simulink model "Logic"  (R2017a)
settings: Solver=FixedStepDiscrete  StartTime=0.0  StopTime=0.1  FixedStep=2e-6  MaxStep=1e-4  RelTol=1e-3
undefined symbols (not defined in the file): DiscIntNeverNeededParam
libraries: powerlib_meascontrol x1, powerlib x1
settings Model: Creator=mayartmal  LastModifiedBy=mayartmal

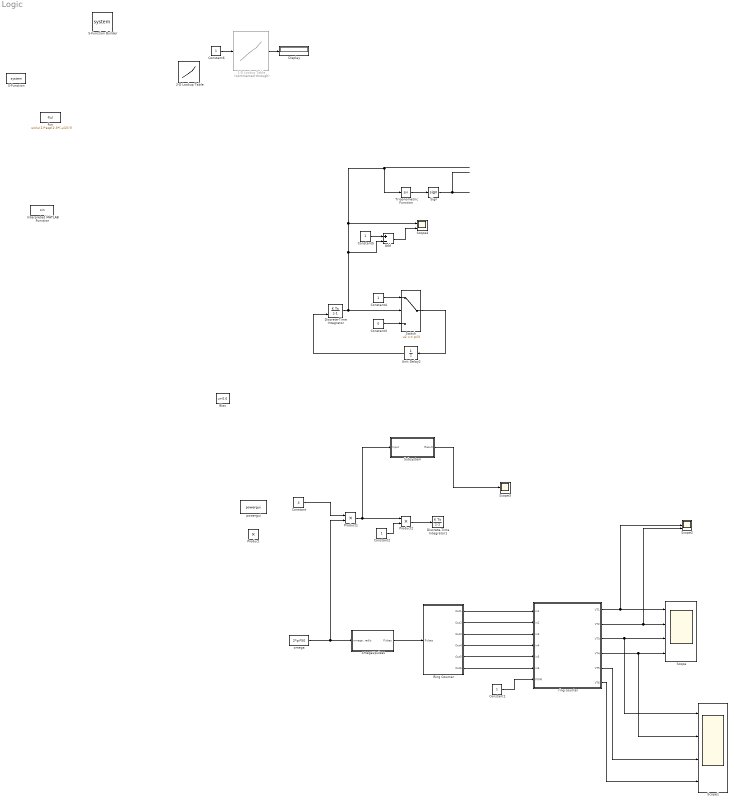
== system Logic ==
  1-D Lookup Table : Lookup_n-D  Commented=through  NumberOfTableDimensions=1  BreakpointsForDimension1=[1:5]  Table=[2:10]  InternalRulePriority=Speed  RndMeth=Simplest  InputSameDT=on
  2-D Lookup Table : Lookup_n-D  BreakpointsForDimension1=[1:3]  BreakpointsForDimension2=[1:3]  InternalRulePriority=Speed  RndMeth=Simplest  InputSameDT=on
  Add : Sum  Inputs=+-
  Bias : Bias  Bias=0.0
  Constant : Constant  Value=4
  Constant{1..2,4..6} (5 alike) : Constant
  Constant3 : Constant  Value=0
  Discrete-Time Integrator : DiscreteIntegrator  gainval=1  ExternalReset=rising  InitialConditionSetting=State (most efficient)  SampleTime=-1  ICPrevOutput=DiscIntNeverNeededParam  ICPrevScaledInput=DiscIntNeverNeededParam
  Discrete-Time Integrator1 : DiscreteIntegrator  gainval=1  InitialConditionSetting=State (most efficient)  SampleTime=-1  ICPrevOutput=DiscIntNeverNeededParam  ICPrevScaledInput=DiscIntNeverNeededParam
  Display : Display
  Fcn : Fcn  Expr=sin(u(1)*exp(2.3*(-u(2))))
  Interpreted MATLAB Function : MATLABFcn
  Product : Product
  Product1 : Product
  Product2 : Product
  Ring Counter : Subsystem
  S-Function : S-Function  SFunctionDeploymentMode=off  EnableBusSupport=off
  S-Function Builder : S-Function  SFunctionDeploymentMode=off  EnableBusSupport=off  mask(S-Function Builder){}
      mask help: Simulink:masks:SFunctionBuilder_MD
      mask init:
      | val = [[.9  0.75 0.75 1 1 .9 .9 1]',[1 1 0.75 0.75 .9 .9 1 .9]'];try , sys = get_param(gcb,'SfunBuilderFcnName');if isempty(sys), sys = get_param(gcb,'FunctionName'); end,catch, sys = get_param(gcb,'FunctionName'); end
      settings: CopyFcn=set_param(gcbh,'LinkStatus','none')  OpenFcn=sfunctionwizard(gcbh)
      mask Display: plot(val(:,1),val(:,2)),disp(sys), port_label('input',1,'u0'), port_label('output',1,'y0')
  Scope : Scope  NumInputPorts=4
  Scope1 : Scope  NumInputPorts=4
  Scope2 : Scope  NumInputPorts=3
  Scope3 : Scope
  Scope4 : Scope  NumInputPorts=2
  Sign : Signum
  Subsystem : Subsystem
  Switch : Switch  Threshold=pi/3
  Trigonometric Function : Trigonometry
  Unit Delay2 : UnitDelay  SampleTime=-1
  omega : Constant  Value=2*pi*50
  omega2pulses : Subsystem
  powergui : powerlib/powergui  Priority=1  SimulationMode=Discrete  SampleTime=2e-6  frequency=60  Iterations=50  frequencyindice=0  Pbase=100e6  ErrMax=1e-4  UnitsV=kV  UnitsW=MW  buscounter=0  FunctionMessages=off  echomessages=off  EnableUseOfTLC=off  CurrentSourceSwitches=off  DisableSnubberDevices=off  DisableRonSwitches=off  DisableVfSwitches=off  DisplayEquations=off  SolverType=Tustin/Backward Euler (TBE)  Interpol=off  ExternalGateDelay=off  methode=off  Ts=100  x0status=blocks  SPID=off  SwTol=0  HookPort=off  RestoreLinks=warning  ResistiveCurrentMeasurement=off  Frange=[0:2:500]  Ylog=off  Xlog=on  ShowGrid=off  save=off  variable=ZData  structure=0  ZoomFFT=off  StartTime=0.0  cycles=1  DisplayStyle=1  fundamental=60  FreqAxis=off  MaxFrequency=1000  frequencyindicesteady=1  RmsSteady=1  display=off
  ring counter : MATLAB Function  TreatAsAtomicUnit=on
  wires:
  omega2pulses/1(Pulses) -> Ring Counter/1(Pulses)
  Constant1/1 -> ring counter/7(PWM)
  ring counter/1(VT1) -> Scope2/2, Scope/1
  Ring Counter/3(Out3) -> ring counter/3(in3)
  Ring Counter/4(Out4) -> ring counter/4(in4)
  Ring Counter/2(Out2) -> ring counter/2(in2)
  Ring Counter/5(Out5) -> ring counter/5(in5)
  Ring Counter/1(Out1) -> ring counter/1(in1)
  Ring Counter/6(Out6) -> ring counter/6(in6)
  ring counter/2(VT2) -> Scope2/3, Scope/2
  ring counter/3(VT3) -> Scope1/1, Scope/3
  ring counter/4(VT4) -> Scope1/2, Scope/4
  ring counter/5(VT5) -> Scope1/3
  ring counter/6(VT6) -> Scope1/4
  omega/1 -> Product1/2, omega2pulses/1("omega, rad/s")
  Constant/1 -> Product1/1
  Discrete-Time Integrator/1 -> Switch/2, Trigonometric Function/1, Scope4/1, Add/2
  Constant5/1 -> Add/1
  Add/1 -> Scope4/2
  Constant3/1 -> Switch/3
  Switch/1 -> Unit Delay2/1
  Constant4/1 -> Switch/1
  Sign/1 -> ?
  Trigonometric Function/1 -> Sign/1
  Unit Delay2/1 -> Discrete-Time Integrator/2
  Product2/1 -> Discrete-Time Integrator1/1
  Product1/1 -> Subsystem/1(Input), Product2/1
  Constant2/1 -> Product2/2
  Subsystem/1(Result) -> Scope3/1
  Constant6/1 -> 1-D Lookup Table/1
  1-D Lookup Table/1 -> Display/1

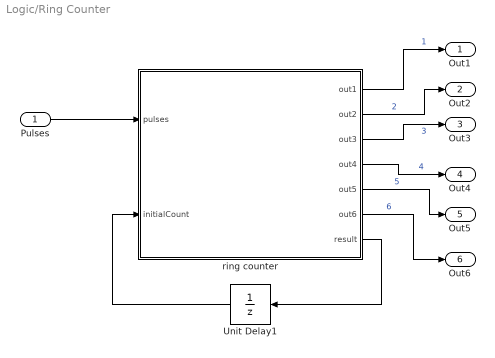
== system Logic/Ring Counter ==
  Pulses : Inport
  Unit Delay1 : UnitDelay  InitialCondition=1  SampleTime=-1
  ring counter : MATLAB Function  TreatAsAtomicUnit=on
  Out1 : Outport
  Out2 : Outport  Port=2
  Out3 : Outport  Port=3
  Out4 : Outport  Port=4
  Out5 : Outport  Port=5
  Out6 : Outport  Port=6
  wires:
  Unit Delay1/1 -> ring counter/2(initialCount)
  ring counter/7(result) -> Unit Delay1/1
  ring counter/3(out3) -> Out3/1  "3"
  ring counter/5(out5) -> Out5/1  "5"
  ring counter/4(out4) -> Out4/1  "4"
  ring counter/2(out2) -> Out2/1  "2"
  ring counter/6(out6) -> Out6/1  "6"
  Pulses/1 -> ring counter/1(pulses)
  ring counter/1(out1) -> Out1/1  "1"

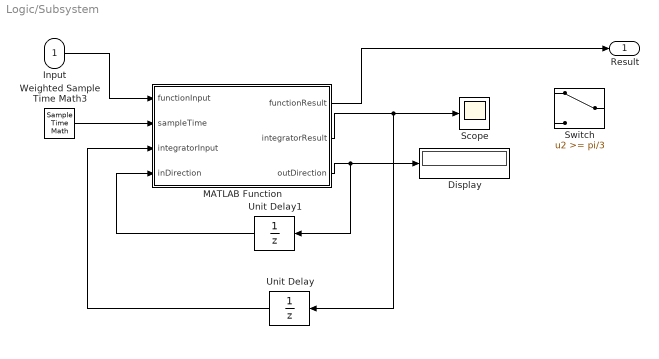
== system Logic/Subsystem ==
  Input : Inport
  Display : Display
  MATLAB Function : MATLAB Function  TreatAsAtomicUnit=on
  Scope : Scope
  Switch : Switch  Threshold=pi/3
  Unit Delay : UnitDelay  SampleTime=-1
  Unit Delay1 : UnitDelay  SampleTime=-1
  Weighted Sample Time Math3 : SampleTimeMath  TsampMathOp=Ts Only
  Result : Outport
  wires:
  Unit Delay/1 -> MATLAB Function/3(integratorInput)
  MATLAB Function/2(integratorResult) -> Scope/1, Unit Delay/1
  MATLAB Function/1(functionResult) -> Result/1
  Weighted Sample Time Math3/1 -> MATLAB Function/2(sampleTime)
  Input/1 -> MATLAB Function/1(functionInput)
  Unit Delay1/1 -> MATLAB Function/4(inDirection)
  MATLAB Function/3(outDirection) -> Unit Delay1/1, Display/1

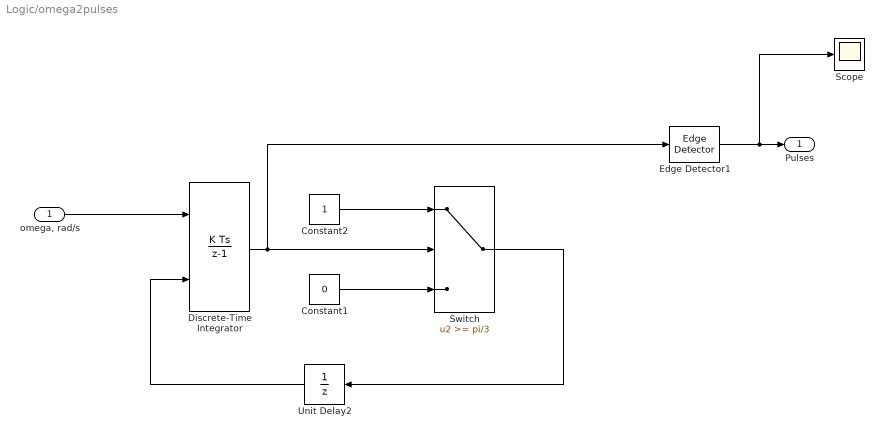
== system Logic/omega2pulses ==
  "omega, rad/s" : Inport
  Constant1 : Constant  Value=0
  Constant2 : Constant
  Discrete-Time Integrator : DiscreteIntegrator  ExternalReset=rising  InitialConditionSetting=State (most efficient)  SampleTime=-1  ICPrevOutput=DiscIntNeverNeededParam  ICPrevScaledInput=DiscIntNeverNeededParam
  Edge Detector1 : powerlib_meascontrol/Logic/Edge Detector  model=Falling  ic=0  Ts=-1
      settings: SourceProductName=Simscape Power Systems  SourceProductBaseCode=PS
  Scope : Scope
  Switch : Switch  Threshold=pi/3
  Unit Delay2 : UnitDelay  SampleTime=-1
  Pulses : Outport
  wires:
  Switch/1 -> Unit Delay2/1
  Discrete-Time Integrator/1 -> Edge Detector1/1, Switch/2
  Unit Delay2/1 -> Discrete-Time Integrator/2
  Constant1/1 -> Switch/3
  Constant2/1 -> Switch/1
  Edge Detector1/1 -> Scope/1, Pulses/1
  "omega, rad/s"/1 -> Discrete-Time Integrator/1

== matlab function Logic/ring counter ==
  data: in1 input; in2 input; in3 input; in4 input; in5 input; in6 input; VT1 output; PWM input; VT2 output; VT3 output; VT4 output; VT5 output; VT6 output
function [VT1, VT2, VT3, VT4, VT5, VT6] = fcn(in1, in2, in3, in4, in5, in6, PWM)

VT1 = in1 | (in2 & PWM) | in3 |(in5 & (~PWM));
VT2 = (in2 & (~PWM)) | in4 | (in5 & PWM) | in6;

VT3 = in3 | (in4 & PWM) | in5 |(in1 & (~PWM));
VT4 = (in4 & (~PWM)) | in6 | (in1 & PWM) | in2;

VT5 = in5 | (in6 & PWM) | in1 |(in3 & (~PWM));
VT6 = (in6 & (~PWM)) | in2 | (in3 & PWM) | in4;



end

== matlab function Logic/Subsystem/MATLAB Function ==
  data: functionResult output; functionInput input; sampleTime input; integratorResult output; integratorInput input; inDirection input; outDirection output
function [functionResult, integratorResult, outDirection]= fcn(functionInput, sampleTime, integratorInput, inDirection)
if inDirection == 0
    integratorResult = integratorInput + sampleTime;
elseif inDirection == 1
    integratorResult = integratorInput - sampleTime;
else
    integratorResult = integratorInput;
end

functionResult = functionInput * integratorResult;

if functionResult >= 10
    outDirection = 1;
elseif functionResult <= 0
    outDirection = 0;
else 
    outDirection = inDirection;
end




end

== matlab function Logic/Ring Counter/ring counter ==
  data: pulses input; out1 output; out2 output; initialCount input; out3 output; out4 output; out5 output; out6 output; result output
function [out1, out2, out3, out4, out5, out6, result] = fcn(pulses, initialCount)
if pulses == 1 
   result = initialCount + 1;
   if result >= 7
       result = 1;
   end        
else   
   result = initialCount;
end

%out1
if result == 1
       out1 = 1;
else
       out1 = 0;
end
%%out2
if result == 2
       out2 = 1;
else
       out2 = 0;
end
%out3
if result == 3
       out3 = 1;
else
       out3 = 0;
end
%out4
if result == 4
       out4 = 1;
else
       out4 = 0;
end
%out5
if result == 5
       out5 = 1;
else
       out5 = 0;
end 
%out6
if result == 6
       out6 = 1;
else
       out6 = 0;
end


end
